simulink model "main"  (R2024b)
settings: Solver=FixedStepAuto  StartTime=0.0  StopTime=5  FixedStep=Ts  RelTol=1e-3
settings Model: Creator=marti  LastModifiedBy=marti
settings DataIOCC: FinalStateName=xf  SaveFinalState=on  SaveOperatingPoint=on

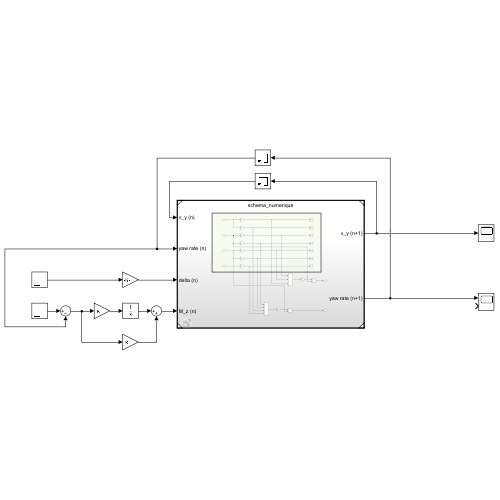
[thumbnail: Simulink's stored preview of the top-level diagram]
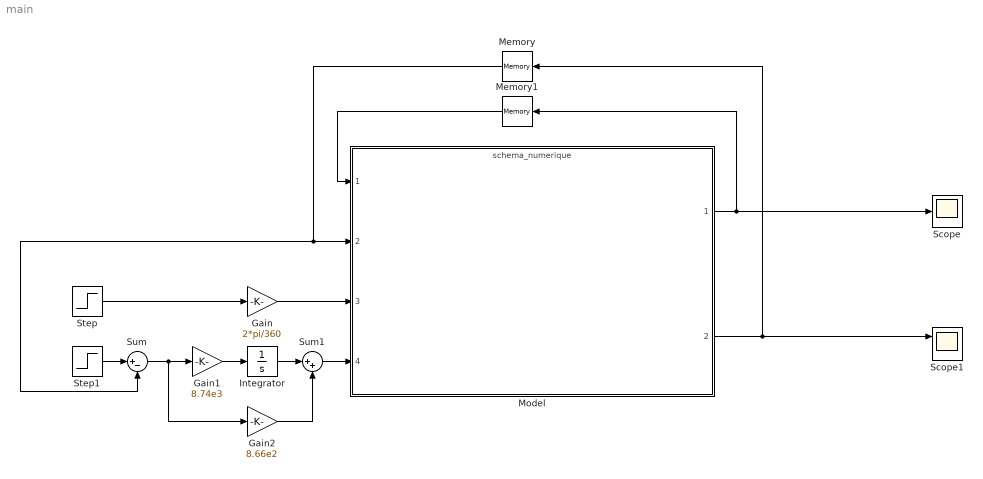
== system main ==
  Gain : Gain  Gain=2*pi/360
  Gain1 : Gain  Gain=8.74e3
  Gain2 : Gain  Gain=8.66e2
  Integrator : Integrator
  Memory : Memory
  Memory1 : Memory
  Model : ModelReference  ModelNameDialog=schema_numerique.slx  SimulationMode=Normal  ModelReferenceVersion=1.3
  Scope : Scope
  Scope1 : Scope  NumInputPorts=2
  Step : Step  After=0  SampleTime=0
  Step1 : Step  SampleTime=0
  Sum : Sum  Inputs=|+-
  Sum1 : Sum  Inputs=|++
  wires:
  Step/1 -> Gain/1
  Model/1 -> Scope/1, Memory1/1
  Memory1/1 -> Model/1
  Memory/1 -> Sum/2, Model/2
  Gain/1 -> Model/3
  Model/2 -> Scope1/1, Memory/1
  Step1/1 -> Sum/1
  Sum/1 -> Gain2/1, Gain1/1
  Gain1/1 -> Integrator/1
  Integrator/1 -> Sum1/1
  Sum1/1 -> Model/4
  Gain2/1 -> Sum1/2
